simulink model "test1"  (R2020b)
settings: Solver=ode1  StartTime=0.0  StopTime=20  FixedStep=0.001  RelTol=1e-3
undefined symbols (not defined in the file): kd, kd_best, ki, ki_best, kp, kp_best, mot, National_Instruments, PCIe, sens
libraries: simulink x20, sldrtlib x3
settings Model: ExtModeTrigDuration=50000  Creator=pellizzar1  LastModifiedBy=pellizzar1
settings DataIOCC: ReturnWorkspaceOutputs=off
settings RTWCC: Description=Simulink Desktop Real-Time  SystemTargetFile=sldrt.tlc  TemplateMakefile=sldrt.tmf  RTWCompilerOptimization=on
settings CodeAppCC: MaxIdLength=95
settings SimulinkDesktopRealTimeCC: TargetPreCompLibLocation=C:\Program Files\MATLAB\R2020b\toolbox\sldrt\lib\win64

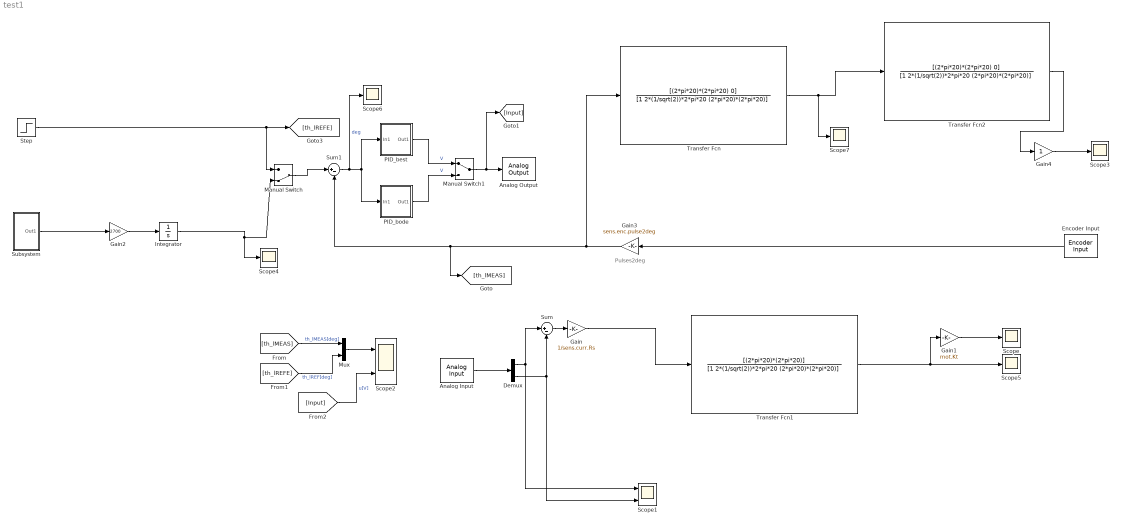
== system test1 ==
  note: Pulses2deg
  Analog Input : sldrtlib/Analog Input  SampleTime=0.001  MaxMissedTicks=10  ShowMissedTicks=off  YieldWhenWaiting=off  DrvName=National_Instruments/PCIe-6321  DrvAddress=4294967295  DrvOptions=[0 0 0 2 0 0 0]  Channels=[1,2]  RangeMode=1  VoltRange=1  DataType=1
      settings: AttributesFormatString=National Instruments\nPCIe-6321 [auto]
  Analog Output : sldrtlib/Analog Output  SampleTime=0.001  MaxMissedTicks=10  ShowMissedTicks=off  YieldWhenWaiting=off  DrvName=National_Instruments/PCIe-6321  DrvAddress=4294967295  DrvOptions=[0 0 0 2 0 0 0]  Channels=1  RangeMode=1  VoltRange=1  InitialValue=0  FinalValue=0
      settings: AttributesFormatString=National Instruments\nPCIe-6321 [auto]
  Demux : Demux  Outputs=2
  Encoder Input : sldrtlib/Encoder Input  SampleTime=0.001  MaxMissedTicks=10  ShowMissedTicks=off  YieldWhenWaiting=off  DrvName=National_Instruments/PCIe-6321  DrvAddress=4294967295  DrvOptions=[0 0 0 2 0 0 0]  Channels=1  QuadMode=3  IndexPulse=1  InputFilter=Inf  DataType=1
      settings: AttributesFormatString=National Instruments\nPCIe-6321 [auto]
  Gain : Gain  Gain=1/sens.curr.Rs
  Gain1 : Gain  Gain=mot.Kt
  Gain2 : Gain  Gain=2700
  Gain3 : Gain  Gain=sens.enc.pulse2deg
  Gain4 : Gain
  Integrator : Integrator
  Manual Switch : ManualSwitch  CurrentSetting=0
  Manual Switch1 : ManualSwitch
  Mux : Mux  Inputs=2
  PID_best : Subsystem
  PID_bode : Subsystem
  Scope{,3..7} (6 alike) : Scope
  Scope1 : Scope  NumInputPorts=2
  Scope2 : Scope  NumInputPorts=2
  Step : Step  After=360  SampleTime=0
  Subsystem : Subsystem
  Sum : Sum  Inputs=|+-
  Sum1 : Sum  Inputs=|+-
  Transfer Fcn : TransferFcn  Numerator=[(2*pi*20)*(2*pi*20) 0]  Denominator=[1 2*(1/sqrt(2))*2*pi*20 (2*pi*20)*(2*pi*20)]
  Transfer Fcn1 : TransferFcn  Numerator=[(2*pi*20)*(2*pi*20)]  Denominator=[1 2*(1/sqrt(2))*2*pi*20 (2*pi*20)*(2*pi*20)]
  Transfer Fcn2 : TransferFcn  Numerator=[(2*pi*20)*(2*pi*20) 0]  Denominator=[1 2*(1/sqrt(2))*2*pi*20 (2*pi*20)*(2*pi*20)]
  wires:
  Analog Input/1 -> Demux/1
  Demux/1 -> Sum/1, Scope1/1
  Demux/2 -> Sum/2, Scope1/2
  Manual Switch1/1 -> [Input], Analog Output/1
  Mux/1 -> Scope2/1
  [th_lREFE] -> Mux/2  "th_lREF[deg]"
  Manual Switch/1 -> Sum1/1
  PID_best/1(Out1) -> Manual Switch1/1  "V"
  [Input] -> Scope2/2  "u[V]"
  [th_lMEAS] -> Mux/1  "th_lMEAS[deg]"
  Gain3/1 -> Transfer Fcn/1, Sum1/2, [th_lMEAS]
  Sum1/1 -> Scope6/1, PID_best/1(In1), PID_bode/1(In1)  "deg"
  PID_bode/1(Out1) -> Manual Switch1/2  "V"
  Step/1 -> Manual Switch/1, [th_lREFE]
  Sum/1 -> Gain/1
  Gain1/1 -> Scope/1
  Gain2/1 -> Integrator/1
  Gain/1 -> Transfer Fcn1/1
  Transfer Fcn1/1 -> Gain1/1, Scope5/1
  Gain4/1 -> Scope3/1
  Integrator/1 -> Scope4/1, Manual Switch/2
  Transfer Fcn2/1 -> Gain4/1
  Transfer Fcn/1 -> Scope7/1, Transfer Fcn2/1
  Encoder Input/1 -> Gain3/1
  Subsystem/1(Out1) -> Gain2/1

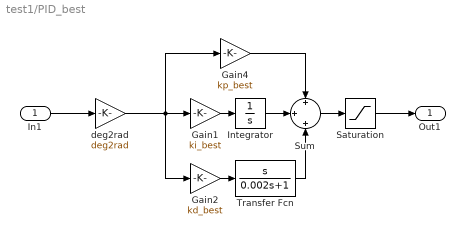
== system test1/PID_best ==
  In1 : Inport
  Gain1 : Gain  Gain=ki_best
  Gain2 : Gain  Gain=kd_best
  Gain4 : Gain  Gain=kp_best
  Integrator : Integrator
  Saturation : Saturate  UpperLimit=10  LowerLimit=-10
  Sum : Sum  Inputs=+|+|+
  Transfer Fcn : TransferFcn  Numerator=[1 0]  Denominator=[0.002 1]
  deg2rad : Gain  Gain=deg2rad
  Out1 : Outport
  wires:
  Transfer Fcn/1 -> Sum/3
  deg2rad/1 -> Gain1/1, Gain4/1, Gain2/1
  In1/1 -> deg2rad/1
  Gain2/1 -> Transfer Fcn/1
  Sum/1 -> Saturation/1
  Saturation/1 -> Out1/1
  Integrator/1 -> Sum/2
  Gain1/1 -> Integrator/1
  Gain4/1 -> Sum/1

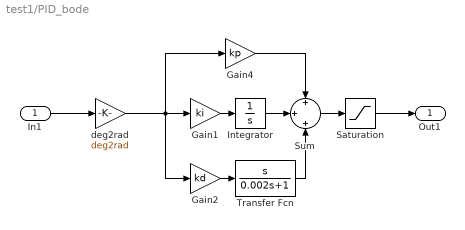
== system test1/PID_bode ==
  In1 : Inport
  Gain1 : Gain  Gain=ki
  Gain2 : Gain  Gain=kd
  Gain4 : Gain  Gain=kp
  Integrator : Integrator
  Saturation : Saturate  UpperLimit=10  LowerLimit=-10
  Sum : Sum  Inputs=+|+|+
  Transfer Fcn : TransferFcn  Numerator=[1 0]  Denominator=[0.002 1]
  deg2rad : Gain  Gain=deg2rad
  Out1 : Outport
  wires:
  Gain4/1 -> Sum/1
  Gain1/1 -> Integrator/1
  Integrator/1 -> Sum/2
  Saturation/1 -> Out1/1
  Sum/1 -> Saturation/1
  Gain2/1 -> Transfer Fcn/1
  In1/1 -> deg2rad/1
  deg2rad/1 -> Gain2/1, Gain4/1, Gain1/1
  Transfer Fcn/1 -> Sum/3

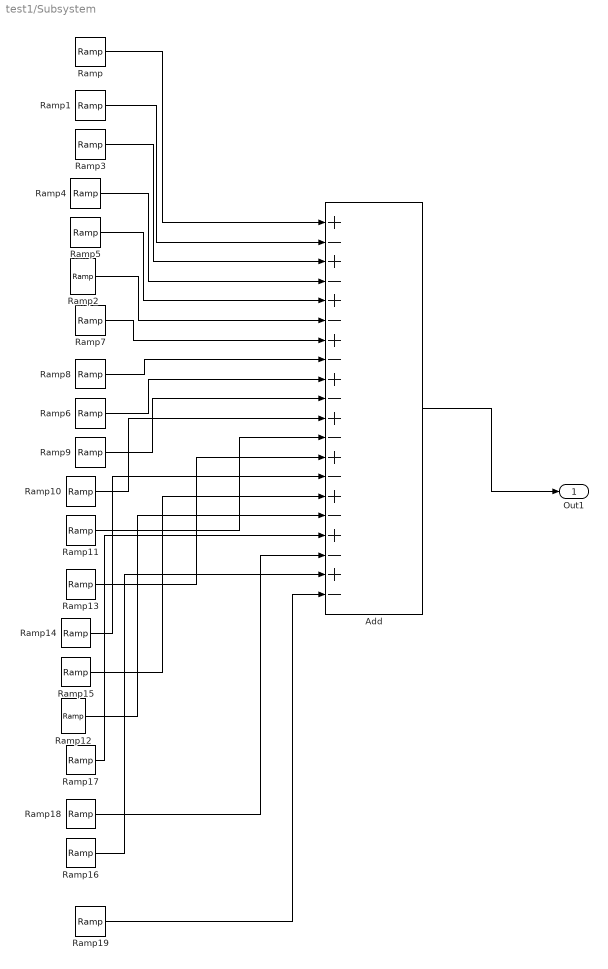
== system test1/Subsystem ==
  Add : Sum  Inputs=+-+-+-+-+-+-+-+-+-+-
  Ramp : simulink/Sources/Ramp  slope=1  start=0  InitialOutput=0
  Ramp1 : simulink/Sources/Ramp  slope=2  start=1  InitialOutput=0
  Ramp10 : simulink/Sources/Ramp  slope=2  start=10  InitialOutput=0
  Ramp11 : simulink/Sources/Ramp  slope=2  start=11  InitialOutput=0
  Ramp12 : simulink/Sources/Ramp  slope=2  start=15  InitialOutput=0
  Ramp13 : simulink/Sources/Ramp  slope=2  start=12  InitialOutput=0
  Ramp14 : simulink/Sources/Ramp  slope=2  start=13  InitialOutput=0
  Ramp15 : simulink/Sources/Ramp  slope=2  start=14  InitialOutput=0
  Ramp16 : simulink/Sources/Ramp  slope=2  start=18  InitialOutput=0
  Ramp17 : simulink/Sources/Ramp  slope=2  start=16  InitialOutput=0
  Ramp18 : simulink/Sources/Ramp  slope=2  start=17  InitialOutput=0
  Ramp19 : simulink/Sources/Ramp  slope=2  start=19  InitialOutput=0
  Ramp2 : simulink/Sources/Ramp  slope=2  start=5  InitialOutput=0
  Ramp3 : simulink/Sources/Ramp  slope=2  start=2  InitialOutput=0
  Ramp4 : simulink/Sources/Ramp  slope=2  start=3  InitialOutput=0
  Ramp5 : simulink/Sources/Ramp  slope=2  start=4  InitialOutput=0
  Ramp6 : simulink/Sources/Ramp  slope=2  start=8  InitialOutput=0
  Ramp7 : simulink/Sources/Ramp  slope=2  start=6  InitialOutput=0
  Ramp8 : simulink/Sources/Ramp  slope=2  start=7  InitialOutput=0
  Ramp9 : simulink/Sources/Ramp  slope=2  start=9  InitialOutput=0
  Out1 : Outport
  wires:
  Add/1 -> Out1/1
  Ramp2/1 -> Add/6
  Ramp5/1 -> Add/5
  Ramp3/1 -> Add/3
  Ramp1/1 -> Add/2
  Ramp6/1 -> Add/9
  Ramp/1 -> Add/1
  Ramp8/1 -> Add/8
  Ramp9/1 -> Add/10
  Ramp4/1 -> Add/4
  Ramp7/1 -> Add/7
  Ramp10/1 -> Add/11
  Ramp11/1 -> Add/12
  Ramp13/1 -> Add/13
  Ramp14/1 -> Add/14
  Ramp15/1 -> Add/15
  Ramp12/1 -> Add/16
  Ramp17/1 -> Add/17
  Ramp18/1 -> Add/18
  Ramp16/1 -> Add/19
  Ramp19/1 -> Add/20
